simulink model "Closed_WithConstant"  (R2023b)
settings: Solver=VariableStepAuto  StartTime=0.0  StopTime=10.0  RelTol=1e-3
values from neighbouring files (symbols this model uses):
  Area = 2.5    [Closed_Loop_with_PID.m]
  b = 0.1    [Closed_Loop_with_PID.m]
  Capacity = 5    [Closed_Loop_with_PID.m]
  Cd = 0.3    [Closed_Loop_with_PID.m]
  G_ratio = 10    [Closed_Loop_with_PID.m]
  J = 0.01    [Closed_Loop_with_PID.m]
  L = 0.5    [Closed_Loop_with_PID.m]
  m_car = 1000    [Closed_Loop_with_PID.m]
  R = 1    [Closed_Loop_with_PID.m]
  R_bat = 0.5    [Closed_Loop_with_PID.m]
  r_tire = 0.3    [Closed_Loop_with_PID.m]
  rho = 1.225    [Closed_Loop_with_PID.m]
libraries: slpidlib x1
settings Model: Creator=mdhel  LastModifiedBy=mdhel

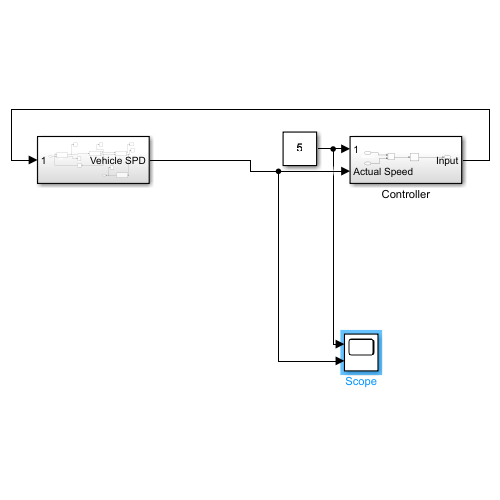
[thumbnail: Simulink's stored preview of the top-level diagram]
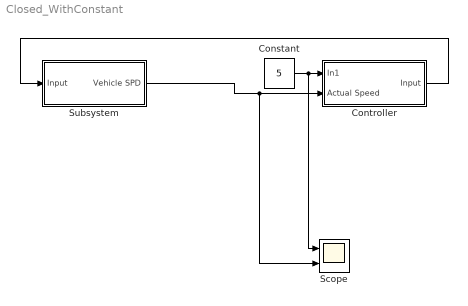
== system Closed_WithConstant ==
  Constant : Constant  Value=5
  Controller : Subsystem
  Scope : Scope  NumInputPorts=2
  Subsystem : Subsystem
  wires:
  Controller/1(Input) -> Subsystem/1(Input)
  Constant/1 -> Scope/1, Controller/1(In1)
  Subsystem/1(Vehicle SPD) -> Scope/2, Controller/2(Actual Speed)

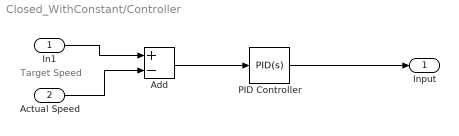
== system Closed_WithConstant/Controller ==
  note: Target Speed
  In1 : Inport
  Actual Speed : Inport  Port=2
  Add : Sum  Inputs=+-
  PID Controller : slpidlib/PID Controller  Controller=PID  Form=Parallel  TimeDomain=Continuous-time  UseExternalTs=off  SampleTime=-1  IntegratorMethod=Forward Euler  FilterMethod=Forward Euler  ControllerParametersSource=internal  P=50  I=25  UseKiTs=off  D=0  N=100  UseFilter=on  TunerSelectOption=Transfer Function Based (PID Tuner App)  InitialConditionSource=internal  InitialConditionForIntegrator=0  InitialConditionForFilter=0  DifferentiatorICPrevScaledInput=0  ExternalReset=none  TrackingMode=off  Kt=1  LimitOutput=off  SatLimitsSource=internal  UpperSaturationLimit=inf  LowerSaturationLimit=-inf  LinearizeAsGain=on  AntiWindupMode=none  Kb=1  LimitIntegrator=off  UpperIntegratorSaturationLimit=inf  LowerIntegratorSaturationLimit=-inf  POutMin=[]  POutMax=[]  IOutMin=[]  IOutMax=[]  DOutMin=[]  DOutMax=[]  NOutMin=[]  NOutMax=[]  SumOutMin=[]  SumOutMax=[]  SaturationOutMin=[]  SaturationOutMax=[]  PParamMin=[]  PParamMax=[]  IParamMin=[]  IParamMax=[]  DParamMin=[]  DParamMax=[]  NParamMin=[]  NParamMax=[]  KbParamMin=[]  KbParamMax=[]  KtParamMin=[]  KtParamMax=[]  KbOutMin=[]  KbOutMax=[]  KtOutMin=[]  KtOutMax=[]  IntegratorOutMin=[]  IntegratorOutMax=[]  FilterOutMin=[]  FilterOutMax=[]  SumI1OutMin=[]  SumI1OutMax=[]  SumI2OutMin=[]  SumI2OutMax=[]  SumI3OutMin=[]  SumI3OutMax=[]  SumI4OutMin=[]  SumI4OutMax=[]  SumDOutMin=[]  SumDOutMax=[]  DifferentiatorOutMin=[]  DifferentiatorOutMax=[]  FilterDiffOutCoefMin=[]  FilterDiffOutCoefMax=[]  ReciprocalOutMin=[]  ReciprocalOutMax=[]  SumDenOutMin=[]  SumDenOutMax=[]  SumNumOutMin=[]  SumNumOutMax=[]  DivideOutMin=[]  DivideOutMax=[]  UdiffTsProdOutMin=[]  UdiffTsProdOutMax=[]  NTsProdOutMin=[]  NTsProdOutMax=[]  UintegralTsProdOutMin=[]  UintegralTsProdOutMax=[]  UngainTsProdOutMin=[]  UngainTsProdOutMax=[]  ClampingZeroOutDataTypeStr=Inherit: Inherit via back propagation  ClampingZeroOutMin=[]  ClampingZeroOutMax=[]  FilterDenConstantOutDataTypeStr=Inherit: Inherit via back propagation  FilterDenConstantOutMin=[]  FilterDenConstantOutMax=[]  PCopyOutDataTypeStr=Inherit: Inherit via back propagation  PCopyOutMin=[]  PCopyOutMax=[]  NCopyOutDataTypeStr=Inherit: Inherit via back propagation  NCopyOutMin=[]  NCopyOutMax=[]  IntegratorContinuousStateAttributes=''  IntegratorStateMustResolveToSignalObject=off  IntegratorRTWStateStorageClass=Auto  FilterContinuousStateAttributes=''  FilterStateMustResolveToSignalObject=off  FilterRTWStateStorageClass=Auto  ParallelPVariant=InternalParameters  IdealPVariant=Disabled  IVariant=InternalParameters  DVariant=InternalParameters  IntegratorVariant=Continuous  SatVariant=Disabled  AWVariant=Passthrough  PCopyVariant=Disabled  TRVariant=Disabled  FdbkBlocksVariant=Forward  IdealPFdbkVariant=Disabled  SatFdbkVariant=Disabled  DerivativeFilterVariant=ContFilter  NVariant=InternalParameters  NCopyVariant=Disabled  FilterICVariant=InternalICsFilter  IntegratorICVariant=InternalICs  ExternalResetVariant=Disabled  TRSumVariant=Passthrough  SumFdbkVariant=Disabled  SumVariant=Sum_PID  TsampFilterVariant=InternalTs  TsampNgainVariant=Passthrough  TsampIntegralVariant=Disabled_SignalSpec  ExternalSaturationOutDataTypeStr=Inherit: Same as second input
  Input : Outport
  wires:
  In1/1 -> Add/1
  Actual Speed/1 -> Add/2
  Add/1 -> PID Controller/1
  PID Controller/1 -> Input/1

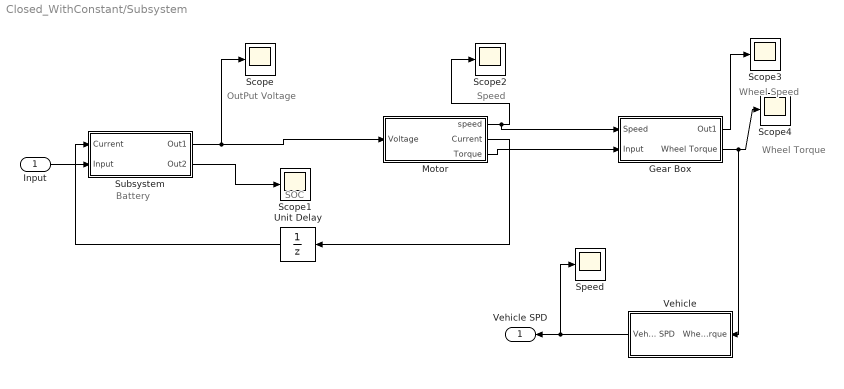
== system Closed_WithConstant/Subsystem ==
  note: SOC
  note: Speed
  note: Wheel Torque
  note: Battery
  note: Wheel Speed
  note: OutPut Voltage
  Input : Inport
  Gear Box : Subsystem
  Motor : Subsystem
  Scope{,1..4} (5 alike) : Scope
  Speed : Scope
  Subsystem : Subsystem
  Unit Delay : UnitDelay  SampleTime=-1  HasFrameUpgradeWarning=on
  Vehicle : Subsystem
  Vehicle SPD : Outport
  wires:
  Gear Box/1(Out1) -> Scope3/1
  Subsystem/1(Out1) -> Motor/1(Voltage), Scope/1
  Unit Delay/1 -> Subsystem/1(Current)
  Motor/3(Torque) -> Gear Box/2(Input)
  Vehicle/1(Vehicle SPD) -> Vehicle SPD/1, Speed/1
  Motor/1(speed) -> Gear Box/1(Speed), Scope2/1
  Gear Box/2(Wheel Torque) -> Vehicle/1(Wheel Torque), Scope4/1
  Subsystem/2(Out2) -> Scope1/1
  Motor/2(Current) -> Unit Delay/1
  Input/1 -> Subsystem/2(Input)

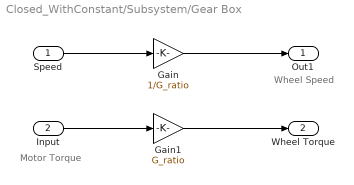
== system Closed_WithConstant/Subsystem/Gear Box ==
  note: Motor Torque
  note: Wheel Speed
  Speed : Inport
  Input : Inport  Port=2
  Gain : Gain  Gain=1/G_ratio
  Gain1 : Gain  Gain=G_ratio
  Out1 : Outport
  Wheel Torque : Outport  Port=2
  wires:
  Speed/1 -> Gain/1
  Gain/1 -> Out1/1
  Input/1 -> Gain1/1
  Gain1/1 -> Wheel Torque/1

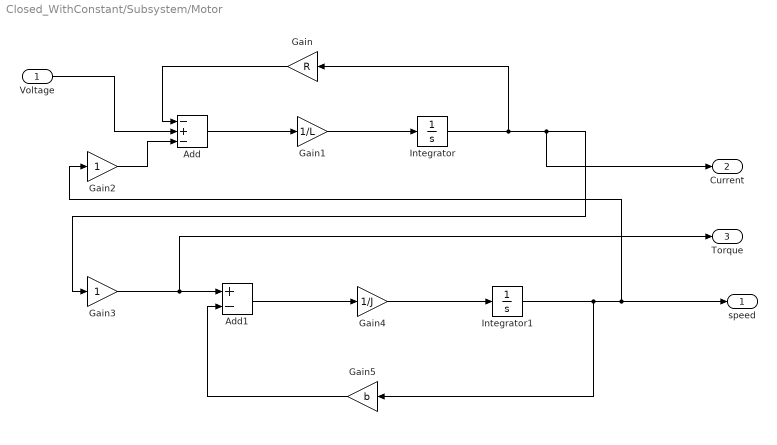
== system Closed_WithConstant/Subsystem/Motor ==
  Voltage : Inport
  Add : Sum  Inputs=-+-
  Add1 : Sum  Inputs=+-
  Gain : Gain  Gain=R
  Gain1 : Gain  Gain=1/L
  Gain2 : Gain
  Gain3 : Gain
  Gain4 : Gain  Gain=1/J
  Gain5 : Gain  Gain=b
  Integrator : Integrator
  Integrator1 : Integrator
  speed : Outport
  Current : Outport  Port=2
  Torque : Outport  Port=3
  wires:
  Voltage/1 -> Add/2
  Gain/1 -> Add/1
  Add/1 -> Gain1/1
  Gain1/1 -> Integrator/1
  Integrator/1 -> Gain/1, Current/1, Gain3/1
  Gain2/1 -> Add/3
  Gain3/1 -> Torque/1, Add1/1
  Add1/1 -> Gain4/1
  Gain4/1 -> Integrator1/1
  Integrator1/1 -> Gain5/1, Gain2/1, speed/1
  Gain5/1 -> Add1/2

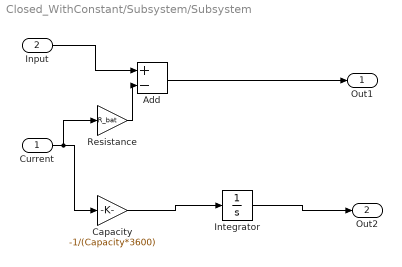
== system Closed_WithConstant/Subsystem/Subsystem ==
  Current : Inport
  Input : Inport  Port=2
  Add : Sum  Inputs=+-
  Capacity : Gain  Gain=-1/(Capacity*3600)
  Integrator : Integrator  InitialCondition=1
  Resistance : Gain  Gain=R_bat
  Out1 : Outport
  Out2 : Outport  Port=2
  wires:
  Input/1 -> Add/1
  Add/1 -> Out1/1
  Capacity/1 -> Integrator/1
  Integrator/1 -> Out2/1
  Current/1 -> Resistance/1, Capacity/1
  Resistance/1 -> Add/2

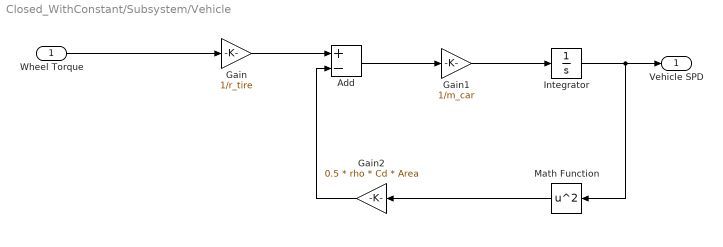
== system Closed_WithConstant/Subsystem/Vehicle ==
  Wheel Torque : Inport
  Add : Sum  Inputs=+-
  Gain : Gain  Gain=1/r_tire
  Gain1 : Gain  Gain=1/m_car
  Gain2 : Gain  Gain=0.5 * rho * Cd * Area
  Integrator : Integrator
  Math Function : Math  Operator=square
  Vehicle SPD : Outport
  wires:
  Wheel Torque/1 -> Gain/1
  Gain/1 -> Add/1
  Add/1 -> Gain1/1
  Gain1/1 -> Integrator/1
  Integrator/1 -> Math Function/1, Vehicle SPD/1
  Gain2/1 -> Add/2
  Math Function/1 -> Gain2/1
